simulink model "Model_TranslationEngine64"  (R2022b)
settings: Solver=FixedStepDiscrete  StartTime=0.0  StopTime=5  RelTol=1e-3  EnableMultiTasking=on
InitFcn:
  | % Initialize model
  | ModelSettings=BTConfig.GetModelSettings();
  | 
  | ModelSettings.Validate();
  | 
  | ModelInit;
  | 
  | 
  | % load library data
  | GainLibrary_data;
  | % Load saved values from partition process
  | CapturedConstMask.LoadMapFromFile(bdroot)
StartFcn:
  | % make sure all the simulated RTC requests are found
  | %RTC_SIM_OBJ.ValidateREQs();
undefined symbols (not defined in the file or in its folder): AA, BPLP, Column, NumHFRefBPF, NumHFRefLPF, NumMusicChannels, Row, VolumeMuteConfig
libraries: TuneVar x925, TOP x490, FeaturePath x111, CapturedConstLib x52
(part 19 of 34)

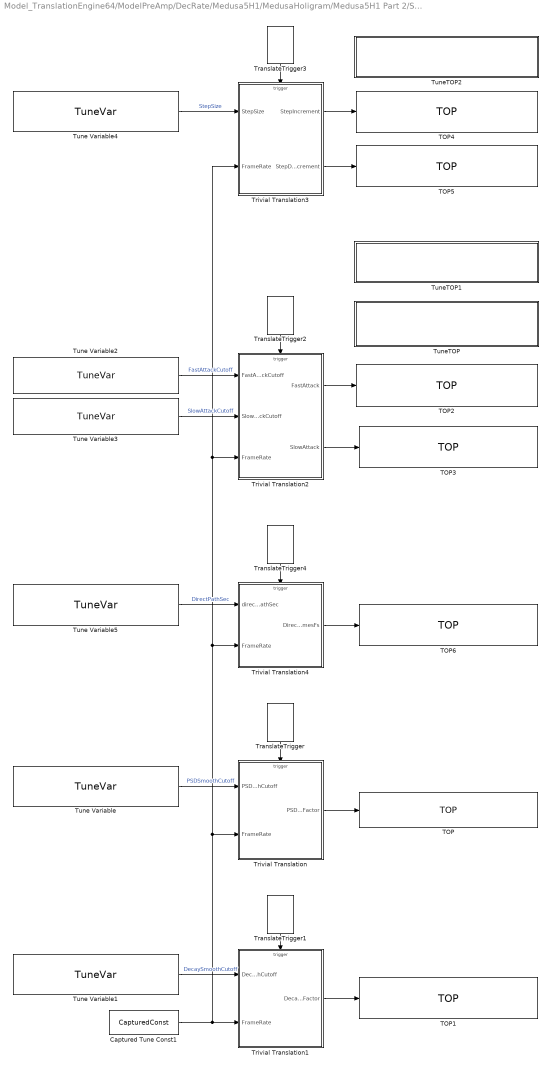
== system Model_TranslationEngine64/ModelPreAmp/DecRate/Medusa5H1/MedusaHoligram/Medusa5H1 Part 2/SPUM Decay Estimate/Decay Estimate ==
  Captured Tune Const1 : CapturedConstLib/CapturedConst  TriggerInit=[-265 -88 -165 -52]  Role=Automatic
      settings: SourceProductName=Bose Talaria
  TOP : TOP/TOP  TriggerInit=[100 -405 360 -355]  TopName=PSDSmoothFactor  DataTypeOut=single  BankNumber=0  PreOverlay=false  PostOverlay=false  Role=Automatic
      settings: SourceProductName=Bose Talaria
  TOP1 : TOP/TOP  TriggerInit=[100 -135 360 -75]  TopName=DecaySmoothFactor  DataTypeOut=single  BankNumber=0  PreOverlay=false  PostOverlay=false  Role=Automatic
      settings: SourceProductName=Bose Talaria
  TOP2 : TOP/TOP  TriggerInit=[95 -1030 360 -970]  TopName=FastAttack  DataTypeOut=single  BankNumber=0  PreOverlay=false  PostOverlay=false  Role=Automatic
      settings: SourceProductName=Bose Talaria
  TOP3 : TOP/TOP  TriggerInit=[100 -940 360 -880]  TopName=SlowAttack  DataTypeOut=single  BankNumber=0  PreOverlay=false  PostOverlay=false  Role=Automatic
      settings: SourceProductName=Bose Talaria
  TOP4 : TOP/TOP  TriggerInit=[95 -1430 360 -1370]  TopName=StepIncrement  DataTypeOut=single  BankNumber=0  PreOverlay=false  PostOverlay=false  Role=Automatic
      settings: SourceProductName=Bose Talaria
  TOP5 : TOP/TOP  TriggerInit=[95 -1350 360 -1290]  TopName=StepDecrement  DataTypeOut=single  BankNumber=0  PreOverlay=false  PostOverlay=false  Role=Automatic
      settings: SourceProductName=Bose Talaria
  TOP6 : TOP/TOP  TriggerInit=[100 -680 360 -620]  TopName=DirectPathFramesFs  DataTypeOut=single  BankNumber=0  PreOverlay=false  PostOverlay=false  Role=Automatic
      settings: SourceProductName=Bose Talaria
  TranslateTrigger : TuneVar/TranslateTrigger  TriggerInit=[-34 -535 4 -480]
      settings: SourceProductName=Bose Talaria
  TranslateTrigger1 : TuneVar/TranslateTrigger  TriggerInit=[-34 -255 4 -200]
      settings: SourceProductName=Bose Talaria
  TranslateTrigger2 : TuneVar/TranslateTrigger  TriggerInit=[-34 -1130 4 -1075]
      settings: SourceProductName=Bose Talaria
  TranslateTrigger3 : TuneVar/TranslateTrigger  TriggerInit=[-34 -1525 4 -1470]
      settings: SourceProductName=Bose Talaria
  TranslateTrigger4 : TuneVar/TranslateTrigger  TriggerInit=[-34 -795 4 -740]
      settings: SourceProductName=Bose Talaria
  Trivial Translation : MATLAB Function  TreatAsAtomicUnit=on
  Trivial Translation1 : MATLAB Function  TreatAsAtomicUnit=on
  Trivial Translation2 : MATLAB Function  TreatAsAtomicUnit=on
  Trivial Translation3 : MATLAB Function  TreatAsAtomicUnit=on
  Trivial Translation4 : MATLAB Function  TreatAsAtomicUnit=on
  Tune Variable : TuneVar/TuneVar  Description=Cutoff frequency for single pole averager that smooths energy sequence for decay estimation.  TuneName=PSDSmoothCutoff  SpecifyMaxSize=off  VariableDim=1 (Row)  MaxSize=[1 1]  TunabilityNumber=2  MinValue=[]  MaxValue=[]  TriggerInit=[-405 -444 -165 -386]  MaskValue=3.890381009312922
      settings: SourceProductName=Bose Talaria
  Tune Variable1 : TuneVar/TuneVar  Description=Cutoff frequency for single pole averager that further smooths decay.  TuneName=DecaySmoothCutoff  SpecifyMaxSize=off  VariableDim=1 (Row)  MaxSize=[1 1]  TunabilityNumber=2  MinValue=[]  MaxValue=[]  TriggerInit=[-405 -169 -165 -111]  MaskValue=0.13777233653605728
      settings: SourceProductName=Bose Talaria
  Tune Variable2 : TuneVar/TuneVar  Description=Cutoff frequency for single pole averager when decay parameter is increasing.  TuneName=FastAttackCutoff  SpecifyMaxSize=off  VariableDim=1 (Row)  MaxSize=[1 1]  TunabilityNumber=2  MinValue=[]  MaxValue=[]  TriggerInit=[-405 -1041 -165 -989]  MaskValue=8.8214110578435392
      settings: SourceProductName=Bose Talaria
  Tune Variable3 : TuneVar/TuneVar  Description=Cutoff frequency for single pole averager when decay parameter is decreasing (slow decay).  TuneName=SlowAttackCutoff  SpecifyMaxSize=off  VariableDim=1 (Row)  MaxSize=[1 1]  TunabilityNumber=2  MinValue=[]  MaxValue=[]  TriggerInit=[-405 -981 -165 -929]  MaskValue=0.27692922573026191
      settings: SourceProductName=Bose Talaria
  Tune Variable4 : TuneVar/TuneVar  Description=Step size for decay slewing.  TuneName=StepSize  SpecifyMaxSize=off  VariableDim=1 (Row)  MaxSize=[1 1]  TunabilityNumber=1  MinValue=[]  MaxValue=[]  TriggerInit=[-405 -1429 -165 -1371]  MaskValue=2
      settings: SourceProductName=Bose Talaria
  Tune Variable5 : TuneVar/TuneVar  Description=This is the time in seconds that separates dry (or direct) and reverb parts. The larger directPathSec becomes, the more energy goes into the “impulse” because a longer period of time past “onset” is considered direct energy. Ideally this value is equivalent to an integer multiple of a frame period.  TuneName=DirectPathSec  SpecifyMaxSize=off  VariableDim=1 (Row)  MaxSize=[1 1]  TunabilityNumber=2  MinValue=[]  MaxValue=[]  TriggerInit=[-405 -710 -165 -650]  MaskValue=0.023219954648526078
      settings: SourceProductName=Bose Talaria
  TuneTOP : Subsystem  Description=Prevent spurious change in slope estimation. Signal energy must overcome the noise floor before we accept current derivative as slope of the decay.  mask(Talaria Trivial Tune TOP){TriggerInit=[95 -1121 360 -1059], TopName=NoiseFloor, TuneName=NoiseFloor, DataTypeOut=single, MaskValue=3, TunabilityNumber=2, MinValue=[], MaxValue=[], BankNumber=0, PreOverlay=false, PostOverlay=false, UseSameName=on}
      mask prompts: TriggerInit "Hidden: MoveFcn redraw"; TopName "Name:"; TuneName "Name of TuneVar:"; DataTypeOut "Data type:"; MaskValue "Default Value:"; TunabilityNumber "Tunability:"; MinValue "Min Value:"; MaxValue "Max Value:"; BankNumber "Target memory bank number:"; PreOverlay "Requires pre-overlay action:"; PostOverlay "Requires post-overlay action:"; UseSameName "Use same name for tune variable and TOP"
      mask help: The TuneTOP block encapsultes a Target Overlay Parameter, a Tune Variable, and a Trivial Translation between them.
      mask init:
      | [ok,activeTopPath,activeTunePath] = TuneTOP_Mask.Init(gcbh);
      settings: MoveFcn=TuneTOP_Mask.CB_TriggerInit(gcbh);
      mask Callback TriggerInit: TuneTOP_Mask.CB_TriggerInit(gcbh);
      mask TypeOptions TopName: TOP/TopName
      mask TypeOptions TuneName: Tune Variable/TuneName
      mask TypeOptions DataTypeOut: TOP/DataTypeOut
      mask TypeOptions MaskValue: Tune Variable/MaskValue
      mask TypeOptions TunabilityNumber: Tune Variable/TunabilityNumber
      mask Callback TunabilityNumber: TuneVarMask.CB_TunabilityNumber(gcbh);
      mask TypeOptions MinValue: Tune Variable/MinValue
      mask TypeOptions MaxValue: Tune Variable/MaxValue
      mask TypeOptions BankNumber: TOP/BankNumber
      mask TypeOptions PreOverlay: TOP/PreOverlay
      mask TypeOptions PostOverlay: TOP/PostOverlay
      mask Callback UseSameName: TuneTOP_Mask.CB_UseSameName(gcbh);
      mask DialogControl toolPanel Prompt: Tuning Tool Hints
      mask DialogControl DescriptionGroup Prompt: Description
      mask DialogControl EditDescription Prompt: Edit Description
      mask DialogControl EditDescription Callback: TuneTOP_Mask.CB_EditDescription(gcbh);
      mask DialogControl TunabilityText Prompt: Easy: Changes nearly every tuning.
      mask DialogControl AdvancedPanel Prompt: Advanced
      mask DialogControl ConvertToFullTranslation Prompt: Irreversible conversion to full translation
      mask DialogControl ConvertToFullTranslation Callback: TuneTOP_Mask.CB_ConvertToFullTranslation(gcbh);
      mask DialogControl ErrorContainer Prompt: Error Messages
      mask Display:
      | % retrieve icon definition
      | [path,w,h] = TuneTOP_Mask.Icon();
      | 
      | % retrieve the block's pixel size
      | pos = get(gcbh,'position');
      | bw = pos(3) - pos(1);
      | bh = pos(4) - pos(2);
      | 
      | % draw centered icon
      | xAdj = bw/2 - w/2 + 5;
      | yAdj = bh/2 - h/2 + 4;
      | for i=1:length(path)
      | 	patch(path(i).x+xAdj, path(i).y+yAdj, path(i).rgb);
      | end
      | 
      | % show the top name or an X
      | if (exist('ok','var') && ok)
      | 	text(bw*0.5, bh*0.2, activeTopPath, 'horizontalAlignment', 'center');
      | 	patch(0,0,[1 1 1]);
      | 	patch(bw,bh,[1 1 1]);
      | else
      | 	tx=bw*0.03;
      | 	ty=bh*0.03;
      | 	patch([0 tx bw bw-tx], [ty 0 bh-ty bh], [1 0 0]);
      | 	patch([0 bw-tx bw tx], [bh-ty 0 ty bh], [1 0 0]);
      | end
  TuneTOP1 : Subsystem  Description=Thresold for detecting an onset strike.  mask(Talaria Trivial Tune TOP){TriggerInit=[95 -1208 360 -1152], TopName=OnsetThreshold, TuneName=OnsetThreshold, DataTypeOut=single, MaskValue=1.875, TunabilityNumber=2, MinValue=[], MaxValue=[], BankNumber=0, PreOverlay=false, PostOverlay=false, UseSameName=on}
      mask prompts: TriggerInit "Hidden: MoveFcn redraw"; TopName "Name:"; TuneName "Name of TuneVar:"; DataTypeOut "Data type:"; MaskValue "Default Value:"; TunabilityNumber "Tunability:"; MinValue "Min Value:"; MaxValue "Max Value:"; BankNumber "Target memory bank number:"; PreOverlay "Requires pre-overlay action:"; PostOverlay "Requires post-overlay action:"; UseSameName "Use same name for tune variable and TOP"
      mask help: The TuneTOP block encapsultes a Target Overlay Parameter, a Tune Variable, and a Trivial Translation between them.
      mask init:
      | [ok,activeTopPath,activeTunePath] = TuneTOP_Mask.Init(gcbh);
      settings: MoveFcn=TuneTOP_Mask.CB_TriggerInit(gcbh);
      mask Callback TriggerInit: TuneTOP_Mask.CB_TriggerInit(gcbh);
      mask TypeOptions TopName: TOP/TopName
      mask TypeOptions TuneName: Tune Variable/TuneName
      mask TypeOptions DataTypeOut: TOP/DataTypeOut
      mask TypeOptions MaskValue: Tune Variable/MaskValue
      mask TypeOptions TunabilityNumber: Tune Variable/TunabilityNumber
      mask Callback TunabilityNumber: TuneVarMask.CB_TunabilityNumber(gcbh);
      mask TypeOptions MinValue: Tune Variable/MinValue
      mask TypeOptions MaxValue: Tune Variable/MaxValue
      mask TypeOptions BankNumber: TOP/BankNumber
      mask TypeOptions PreOverlay: TOP/PreOverlay
      mask TypeOptions PostOverlay: TOP/PostOverlay
      mask Callback UseSameName: TuneTOP_Mask.CB_UseSameName(gcbh);
      mask DialogControl toolPanel Prompt: Tuning Tool Hints
      mask DialogControl DescriptionGroup Prompt: Description
      mask DialogControl EditDescription Prompt: Edit Description
      mask DialogControl EditDescription Callback: TuneTOP_Mask.CB_EditDescription(gcbh);
      mask DialogControl TunabilityText Prompt: Easy: Changes nearly every tuning.
      mask DialogControl AdvancedPanel Prompt: Advanced
      mask DialogControl ConvertToFullTranslation Prompt: Irreversible conversion to full translation
      mask DialogControl ConvertToFullTranslation Callback: TuneTOP_Mask.CB_ConvertToFullTranslation(gcbh);
      mask DialogControl ErrorContainer Prompt: Error Messages
      mask Display:
      | % retrieve icon definition
      | [path,w,h] = TuneTOP_Mask.Icon();
      | 
      | % retrieve the block's pixel size
      | pos = get(gcbh,'position');
      | bw = pos(3) - pos(1);
      | bh = pos(4) - pos(2);
      | 
      | % draw centered icon
      | xAdj = bw/2 - w/2 + 5;
      | yAdj = bh/2 - h/2 + 4;
      | for i=1:length(path)
      | 	patch(path(i).x+xAdj, path(i).y+yAdj, path(i).rgb);
      | end
      | 
      | % show the top name or an X
      | if (exist('ok','var') && ok)
      | 	text(bw*0.5, bh*0.2, activeTopPath, 'horizontalAlignment', 'center');
      | 	patch(0,0,[1 1 1]);
      | 	patch(bw,bh,[1 1 1]);
      | else
      | 	tx=bw*0.03;
      | 	ty=bh*0.03;
      | 	patch([0 tx bw bw-tx], [ty 0 bh-ty bh], [1 0 0]);
      | 	patch([0 bw-tx bw tx], [bh-ty 0 ty bh], [1 0 0]);
      | end
  TuneTOP2 : Subsystem  Description=Threshold to accept change in decay.  mask(Talaria Trivial Tune TOP){TriggerInit=[95 -1508 360 -1452], TopName=SlewThreshold, TuneName=SlewThreshold, DataTypeOut=single, MaskValue=0.8, TunabilityNumber=2, MinValue=[], MaxValue=[], BankNumber=0, PreOverlay=false, PostOverlay=false, UseSameName=on}
      mask prompts: TriggerInit "Hidden: MoveFcn redraw"; TopName "Name:"; TuneName "Name of TuneVar:"; DataTypeOut "Data type:"; MaskValue "Default Value:"; TunabilityNumber "Tunability:"; MinValue "Min Value:"; MaxValue "Max Value:"; BankNumber "Target memory bank number:"; PreOverlay "Requires pre-overlay action:"; PostOverlay "Requires post-overlay action:"; UseSameName "Use same name for tune variable and TOP"
      mask help: The TuneTOP block encapsultes a Target Overlay Parameter, a Tune Variable, and a Trivial Translation between them.
      mask init:
      | [ok,activeTopPath,activeTunePath] = TuneTOP_Mask.Init(gcbh);
      settings: MoveFcn=TuneTOP_Mask.CB_TriggerInit(gcbh);
      mask Callback TriggerInit: TuneTOP_Mask.CB_TriggerInit(gcbh);
      mask TypeOptions TopName: TOP/TopName
      mask TypeOptions TuneName: Tune Variable/TuneName
      mask TypeOptions DataTypeOut: TOP/DataTypeOut
      mask TypeOptions MaskValue: Tune Variable/MaskValue
      mask TypeOptions TunabilityNumber: Tune Variable/TunabilityNumber
      mask Callback TunabilityNumber: TuneVarMask.CB_TunabilityNumber(gcbh);
      mask TypeOptions MinValue: Tune Variable/MinValue
      mask TypeOptions MaxValue: Tune Variable/MaxValue
      mask TypeOptions BankNumber: TOP/BankNumber
      mask TypeOptions PreOverlay: TOP/PreOverlay
      mask TypeOptions PostOverlay: TOP/PostOverlay
      mask Callback UseSameName: TuneTOP_Mask.CB_UseSameName(gcbh);
      mask DialogControl toolPanel Prompt: Tuning Tool Hints
      mask DialogControl DescriptionGroup Prompt: Description
      mask DialogControl EditDescription Prompt: Edit Description
      mask DialogControl EditDescription Callback: TuneTOP_Mask.CB_EditDescription(gcbh);
      mask DialogControl TunabilityText Prompt: Easy: Changes nearly every tuning.
      mask DialogControl AdvancedPanel Prompt: Advanced
      mask DialogControl ConvertToFullTranslation Prompt: Irreversible conversion to full translation
      mask DialogControl ConvertToFullTranslation Callback: TuneTOP_Mask.CB_ConvertToFullTranslation(gcbh);
      mask DialogControl ErrorContainer Prompt: Error Messages
      mask Display:
      | % retrieve icon definition
      | [path,w,h] = TuneTOP_Mask.Icon();
      | 
      | % retrieve the block's pixel size
      | pos = get(gcbh,'position');
      | bw = pos(3) - pos(1);
      | bh = pos(4) - pos(2);
      | 
      | % draw centered icon
      | xAdj = bw/2 - w/2 + 5;
      | yAdj = bh/2 - h/2 + 4;
      | for i=1:length(path)
      | 	patch(path(i).x+xAdj, path(i).y+yAdj, path(i).rgb);
      | end
      | 
      | % show the top name or an X
      | if (exist('ok','var') && ok)
      | 	text(bw*0.5, bh*0.2, activeTopPath, 'horizontalAlignment', 'center');
      | 	patch(0,0,[1 1 1]);
      | 	patch(bw,bh,[1 1 1]);
      | else
      | 	tx=bw*0.03;
      | 	ty=bh*0.03;
      | 	patch([0 tx bw bw-tx], [ty 0 bh-ty bh], [1 0 0]);
      | 	patch([0 bw-tx bw tx], [bh-ty 0 ty bh], [1 0 0]);
      | end
  wires:
  Trivial Translation3/2(StepDecrement) -> TOP5/1
  Trivial Translation3/1(StepIncrement) -> TOP4/1
  Tune Variable4/1 -> Trivial Translation3/1(StepSize)  "StepSize"
  TranslateTrigger3/1 -> Trivial Translation3/Trigger
  Trivial Translation2/2(SlowAttack) -> TOP3/1
  Tune Variable3/1 -> Trivial Translation2/2(SlowAttackCutoff)  "SlowAttackCutoff"
  Tune Variable2/1 -> Trivial Translation2/1(FastAttackCutoff)  "FastAttackCutoff"
  TranslateTrigger2/1 -> Trivial Translation2/Trigger
  Trivial Translation2/1(FastAttack) -> TOP2/1
  Tune Variable1/1 -> Trivial Translation1/1(DecaySmoothCutoff)  "DecaySmoothCutoff"
  TranslateTrigger1/1 -> Trivial Translation1/Trigger
  Trivial Translation1/1(DecaySmoothFactor) -> TOP1/1
  Trivial Translation/1(PSDSmoothFactor) -> TOP/1
  TranslateTrigger/1 -> Trivial Translation/Trigger
  Tune Variable/1 -> Trivial Translation/1(PSDSmoothCutoff)  "PSDSmoothCutoff"
  TranslateTrigger4/1 -> Trivial Translation4/Trigger
  Trivial Translation4/1(DirectPathFramesFs) -> TOP6/1
  Tune Variable5/1 -> Trivial Translation4/1(directPathSec)  "DirectPathSec"
  Captured Tune Const1/1 -> Trivial Translation1/2(FrameRate), Trivial Translation3/2(FrameRate), Trivial Translation2/3(FrameRate), Trivial Translation4/2(FrameRate), Trivial Translation/2(FrameRate)

== system Model_TranslationEngine64/ModelPreAmp/DecRate/Medusa5H1/MedusaHoligram/Medusa5H1 Part 2/SPUM Decay Estimate/High-pass filter > 6kHz ==
  InnerLink : Subsystem  mask(Bose Pool IIR Tunable){FeatureName=HPF, Config=InnerLinkConfig}
      mask prompts: FeatureName "Filter name/purpose"; Config "PoolIirTunableConfig"
      mask help:
      | Pool IIR Tunable is a configurable multi-channel IIR filter that supports one or more channels. This block offers flexibility of tuning the number of stages and coefficients. Different filter coefficients and number of stages (biquads) can be used for each channel filter. The Pool IIR Tunable block supports different implementations, which could be configured at build-time:
      |
      | (i)   Generic: IIR filter code not optimized for any processor
      | (ii)  SharcCore: IIR filters executing on core (uses pooliir.asm CRL)
      | (iii) SharcGulAccel: IIR filters executing on IIR hardware accelerator, offloading MIPS usage from core
      | (iv) SharcGxpAccel: IIR filters take advantage of additional accelerators available on GXP processor
      | (v)  Hexagon: TBD
      |
      | NOTE: When using Pool IIR for Sharc-plus based processors, the codeWorkMemory buffer and input buffer should always be mapped to L1 memory to optimize MIPS utilization and avoid audio artifacts.
      |
      | For more information, please see 'Help'.
      mask init:
      | blkh=gcbh;
      | Config=BTConfig.Assert(blkh,Config);
      | 
      | Config.Validate();
      | Config.DoMaskInit(blkh);
      mask Help:
      | <b>Input signals: </b>
      | AudioIn: input channels [frame size x number of channels]
      | 
      | <b>Output signals: </b>
      | AudioOut: output channels [frame size x number of channels]
      | 
      | <b>Mask parameters: </b>
      | PoolIirTunableConfig
      | Filter name/purpose
      mask TypeOptions FeatureName: PoolIirTunableWithReset/FeatureName
      mask Display: DrawPoolIirIcon;

== system Model_TranslationEngine64/ModelPreAmp/DecRate/Medusa5H1/MedusaHoligram/Medusa5H1 Part 3/On/Delay Tuning ==
  Delay Translation : Subsystem  mask(Alignment Delay Translation){Config=ConfigBTC.AlignmentDelayTranslation}
      mask prompts: Config "MedusaAlignmentDelayTranslationConfig"
      mask help: This block accepts Wiggle Delay and Holigram Filter Delay and outputs all Medusa fixed alignment delay amounts in samples.
      mask init:
      | blkh=gcbh;
      | Config=BTConfig.Assert(blkh,Config);
      | 
      | Config.Validate();
  Tune Variable : TuneVar/TuneVar  TuneName=DeciRateWiggleFilterDelaySamples1  SpecifyMaxSize=off  VariableDim=1 (Row)  MaxSize=[1 1]  TunabilityNumber=1  MinValue=[]  MaxValue=[]  TriggerInit=[-115 25 55 75]  MaskValue=ConfigBTC.AlignmentDelayTranslation.DefaultTuning.DeciRateWiggleDelay
      settings: SourceProductName=Bose Talaria
  Tune Variable1 : TuneVar/TuneVar  TuneName=DeciRateNearWiggleFilterDelaySamples1  SpecifyMaxSize=off  VariableDim=1 (Row)  MaxSize=[1 1]  TunabilityNumber=1  MinValue=[]  MaxValue=[]  TriggerInit=[-115 87 55 133]  MaskValue=ConfigBTC.AlignmentDelayTranslation.DefaultTuning.DeciRateNearWiggleDelay
      settings: SourceProductName=Bose Talaria
  wires:
  Tune Variable1/1 -> Delay Translation/2(DeciRateNearWiggleDelaySamples)  "DeciRateNearWiggleFilterDelaySamples1"
  Tune Variable/1 -> Delay Translation/1(DeciRateWiggleDelaySamples)  "DeciRateWiggleFilterDelaySamples1"

== system Model_TranslationEngine64/ModelPreAmp/DecRate/Medusa5H1/MedusaHoligram/Medusa5H1 Part 3/On/Expand Tail Components ==
  Tail Component EQ : Subsystem  LoadFcn="fprintf(\"\\n ''%s'' block does not support BTC and hence, it will be deprecated soon. Please replace all the active instances of \"\"PooliirwithNonTrivialTranslations\"\" with an equivalent BTC block.\", gcb);"  mask(Bose Pool IIR){maxNumStages=config.tailCompEQ.maxNumStages, numStages=config.tailCompEQ.numStages, sosCoefficients=config.tailCompEQ.coeffs, alias='Default', variantType='Hexagon', FeatureName=tailCompEQ}
      mask prompts: maxNumStages "Maximum number of stages"; numStages "Number of stages per channel"; sosCoefficients "Coefficient pool"; variantType "Variant"; FeatureName "Filter name/purpose"
      mask init: same as Model_TranslationEngine64/ModelPreAmp/DecRate/AudioPilot35/EntertainmentLevelDetection/PreProcessing/PreEmphasisShelfFilter
      mask TypeOptions FeatureName: InnerLink/FeatureName
      mask Display:
      | [path,w,h] = IconIIR_Mask();
      | 
      | % work in pixels since the icon does not scale
      | pos = get(gcbh,'position');
      | bw = pos(3) - pos(1);
      | bh = pos(4) - pos(2);
      | 
      | % Draw centered icon
      | xAdj = bw/2 - w/2;
      | yAdj = bh/2 - h/2 + 4;
      | for i=1:length(path)
      | %     patch(path(i).x+xAdj, path(i).y+yAdj, path(i).rgb);
      |     plot(path(i).x+xAdj, path(i).y+yAdj);
      | end
      | 
      | % Anchor the corners of the coordinate system
      | patch(0,0,[1 1 1]);
      | patch(bw,bh,[1 1 1]);
      | 
      | % Display some text
      | text(bw/2, 1,'Pool IIR', ...
      |     'horizontalAlignment','center', ...
      |     'VerticalAlignment','bottom');
  TuneTOP : Subsystem  mask(Talaria Trivial Tune TOP){TriggerInit=[265 167 435 223], TopName=WiggleFilter, TuneName=WiggleFilter, DataTypeOut=single, MaskValue=config.wiggleFilterDefault, TunabilityNumber=1, MinValue=[], MaxValue=[], BankNumber=0, PreOverlay=false, PostOverlay=false, UseSameName=on}
      mask prompts: TriggerInit "Hidden: MoveFcn redraw"; TopName "Name:"; TuneName "Name of TuneVar:"; DataTypeOut "Data type:"; MaskValue "Default Value:"; TunabilityNumber "Tunability:"; MinValue "Min Value:"; MaxValue "Max Value:"; BankNumber "Target memory bank number:"; PreOverlay "Requires pre-overlay action:"; PostOverlay "Requires post-overlay action:"; UseSameName "Use same name for tune variable and TOP"
      mask help: The TuneTOP block encapsultes a Target Overlay Parameter, a Tune Variable, and a Trivial Translation between them.
      mask init:
      | [ok,activeTopPath,activeTunePath] = TuneTOP_Mask.Init(gcbh);
      settings: MoveFcn=TuneTOP_Mask.CB_TriggerInit(gcbh);
      mask Callback TriggerInit: TuneTOP_Mask.CB_TriggerInit(gcbh);
      mask TypeOptions TopName: TOP/TopName
      mask TypeOptions TuneName: Tune Variable/TuneName
      mask TypeOptions DataTypeOut: TOP/DataTypeOut
      mask TypeOptions MaskValue: Tune Variable/MaskValue
      mask TypeOptions TunabilityNumber: Tune Variable/TunabilityNumber
      mask Callback TunabilityNumber: TuneVarMask.CB_TunabilityNumber(gcbh);
      mask TypeOptions MinValue: Tune Variable/MinValue
      mask TypeOptions MaxValue: Tune Variable/MaxValue
      mask TypeOptions BankNumber: TOP/BankNumber
      mask TypeOptions PreOverlay: TOP/PreOverlay
      mask TypeOptions PostOverlay: TOP/PostOverlay
      mask Callback UseSameName: TuneTOP_Mask.CB_UseSameName(gcbh);
      mask DialogControl toolPanel Prompt: Tuning Tool Hints
      mask DialogControl DescriptionGroup Prompt: Description
      mask DialogControl EditDescription Prompt: Edit Description
      mask DialogControl EditDescription Callback: TuneTOP_Mask.CB_EditDescription(gcbh);
      mask DialogControl TunabilityText Prompt: Easy: Changes nearly every tuning.
      mask DialogControl AdvancedPanel Prompt: Advanced
      mask DialogControl ConvertToFullTranslation Prompt: Irreversible conversion to full translation
      mask DialogControl ConvertToFullTranslation Callback: TuneTOP_Mask.CB_ConvertToFullTranslation(gcbh);
      mask DialogControl ErrorContainer Prompt: Error Messages
      mask DialogControl ErrorText Prompt: Default value cannot be empty. Tune variables must have non-zero dimensions.
      mask Display:
      | % retrieve icon definition
      | [path,w,h] = TuneTOP_Mask.Icon();
      | 
      | % retrieve the block's pixel size
      | pos = get(gcbh,'position');
      | bw = pos(3) - pos(1);
      | bh = pos(4) - pos(2);
      | 
      | % draw centered icon
      | xAdj = bw/2 - w/2 + 5;
      | yAdj = bh/2 - h/2 + 4;
      | for i=1:length(path)
      | 	patch(path(i).x+xAdj, path(i).y+yAdj, path(i).rgb);
      | end
      | 
      | % show the top name or an X
      | if (exist('ok','var') && ok)
      | 	text(bw*0.5, bh*0.2, activeTopPath, 'horizontalAlignment', 'center');
      | 	patch(0,0,[1 1 1]);
      | 	patch(bw,bh,[1 1 1]);
      | else
      | 	tx=bw*0.03;
      | 	ty=bh*0.03;
      | 	patch([0 tx bw bw-tx], [ty 0 bh-ty bh], [1 0 0]);
      | 	patch([0 bw-tx bw tx], [bh-ty 0 ty bh], [1 0 0]);
      | end

== system Model_TranslationEngine64/ModelPreAmp/DecRate/Medusa5H1/MedusaHoligram/Medusa5H1 Part 3/On/Full-rate Mixer ==
  Full-Rate Mixer with CAE & Fade Ramper : Subsystem  mask{MedusaFRMConfig=config.FRMConfig, MedusaFRMTune=config.FRMTune}
      mask prompts: MedusaFRMConfig "Config struct name:"; MedusaFRMTune "Tune struct name:"
      mask init:
      | %MedusaConfig = generateMedusaConfig(system_definitions);
      | 
      | % Initialize model parameters
      | %MedusaFullRateMixerInit(MedusaConfig);

== system Model_TranslationEngine64/ModelPreAmp/DecRate/Medusa5H1/MedusaHoligram/Medusa5H1 Part 3/On/Premix ==
  Premix with Mono-Surround & CAE with Fade Ramper : Subsystem  mask(Medusa Premix 5H){MedusaPremixConfig=config.PremixConfig, MedusaPremixTune=config.PremixTune, MSConfig=config.MSConfig}
      mask prompts: MedusaPremixConfig "Config struct name:"; MedusaPremixTune "Tune struct name:"; MSConfig "Mono-Surround Config:"
      mask init:
      | % RTC_SIM_OBJ = RTC_SimData();
      | 
      | % MedusaConfig = generateMedusaConfig(system_definitions);
      | 
      | % Initialize model parameters
      | % MedusaPremixExampleInit(MedusaConfig);
      settings: LibrarySourceBlock=MedusaPremix/Premix with Mono-Surround & CAE with Fade Ramper

== system Model_TranslationEngine64/ModelPreAmp/DecRate/Medusa5H1/MedusaHoligram/Medusa5H1 Part 3/On/VLS Gains Computation ==
  VLS Gains Drv : Subsystem  mask(VLS Gains){configStruct=vlsConfigStruct.VLSGainsConfig, tuneStruct=vlsConfigStruct.VLSGainsTune, FeatureName=VLSDrvGains}
      mask prompts: configStruct "Config struct name:"; tuneStruct "Tune struct name:"; FeatureName "FeaturePath name:"
      mask init:
      | VLSGainsMaskInit(gcbh, FeatureName);
      mask TypeOptions FeatureName: FeaturePath/FeatureName
  VLS Gains Pax : Subsystem  mask(VLS Gains){configStruct=vlsConfigStruct.VLSGainsConfig, tuneStruct=vlsConfigStruct.VLSGainsTune, FeatureName=VLSPaxGains}
      mask prompts: configStruct "Config struct name:"; tuneStruct "Tune struct name:"; FeatureName "FeaturePath name:"
      mask init:
      | VLSGainsMaskInit(gcbh, FeatureName);
      mask TypeOptions FeatureName: FeaturePath/FeatureName

== system Model_TranslationEngine64/ModelPreAmp/DecRate/Medusa5H1/MedusaHoligram/Medusa5H1 Part 4/On/DR Mix Matrix with Hybrid Holigram EQ ==
  FeaturePath : FeaturePath/FeaturePath  FeatureName=DRHoligram  IsGroup=off  GroupNumber=-1  IsModule=off  TriggerInit=[375 434 490 541]
      settings: SourceProductName=Bose Talaria
  IIR : Subsystem  mask(Bose Pool IIR Tunable){FeatureName=PoolIirTunableConfig, Config=Config.Iir}
      mask prompts: FeatureName "Filter name/purpose"; Config "PoolIirTunableConfig"
      mask help:
      | Pool IIR Tunable is a configurable multi-channel IIR filter that supports one or more channels. This block offers flexibility of tuning the number of stages and coefficients. Different filter coefficients and number of stages (biquads) can be used for each channel filter. The Pool IIR Tunable block supports different implementations, which could be configured at build-time:
      |
      | (i)   Generic: IIR filter code not optimized for any processor
      | (ii)  SharcCore: IIR filters executing on core (uses pooliir.asm CRL)
      | (iii) SharcGulAccel: IIR filters executing on IIR hardware accelerator, offloading MIPS usage from core
      | (iv) SharcGxpAccel: IIR filters take advantage of additional accelerators available on GXP processor
      | (v)  Hexagon: TBD
      |
      | NOTE: When using Pool IIR for Sharc-plus based processors, the codeWorkMemory buffer and input buffer should always be mapped to L1 memory to optimize MIPS utilization and avoid audio artifacts.
      |
      | For more information, please see 'Help'.
      mask init:
      | blkh=gcbh;
      | Config=BTConfig.Assert(blkh,Config);
      | 
      | Config.Validate();
      | Config.DoMaskInit(blkh);
      mask Help:
      | <b>Input signals: </b>
      | AudioIn: input channels [frame size x number of channels]
      | 
      | <b>Output signals: </b>
      | AudioOut: output channels [frame size x number of channels]
      | 
      | <b>Mask parameters: </b>
      | PoolIirTunableConfig
      | Filter name/purpose
      mask TypeOptions FeatureName: PoolIirTunableWithReset/FeatureName
      mask Display: DrawPoolIirIcon;
  Tune Translations : Subsystem

== system Model_TranslationEngine64/ModelPreAmp/DecRate/Medusa5H1/MedusaHoligram/Medusa5H1 Part 4/On/FR IIR Holigram EQ ==
  FeaturePath : FeaturePath/FeaturePath  FeatureName=FRHoligram  IsGroup=off  GroupNumber=-1  IsModule=off  TriggerInit=[225 439 340 546]
      settings: SourceProductName=Bose Talaria
  IIR : Subsystem  mask(Bose Pool IIR Tunable){FeatureName=IirConfig, Config=IirConfig}
      mask prompts: FeatureName "Filter name/purpose"; Config "PoolIirTunableConfig"
      mask help:
      | Pool IIR Tunable is a configurable multi-channel IIR filter that supports one or more channels. This block offers flexibility of tuning the number of stages and coefficients. Different filter coefficients and number of stages (biquads) can be used for each channel filter. The Pool IIR Tunable block supports different implementations, which could be configured at build-time:
      |
      | (i)   Generic: IIR filter code not optimized for any processor
      | (ii)  SharcCore: IIR filters executing on core (uses pooliir.asm CRL)
      | (iii) SharcGulAccel: IIR filters executing on IIR hardware accelerator, offloading MIPS usage from core
      | (iv) SharcGxpAccel: IIR filters take advantage of additional accelerators available on GXP processor
      | (v)  Hexagon: TBD
      |
      | NOTE: When using Pool IIR for Sharc-plus based processors, the codeWorkMemory buffer and input buffer should always be mapped to L1 memory to optimize MIPS utilization and avoid audio artifacts.
      |
      | For more information, please see 'Help'.
      mask init:
      | blkh=gcbh;
      | Config=BTConfig.Assert(blkh,Config);
      | 
      | Config.Validate();
      | Config.DoMaskInit(blkh);
      mask Help:
      | <b>Input signals: </b>
      | AudioIn: input channels [frame size x number of channels]
      | 
      | <b>Output signals: </b>
      | AudioOut: output channels [frame size x number of channels]
      | 
      | <b>Mask parameters: </b>
      | PoolIirTunableConfig
      | Filter name/purpose
      mask TypeOptions FeatureName: PoolIirTunableWithReset/FeatureName
      mask Display: DrawPoolIirIcon;

== system Model_TranslationEngine64/ModelPreAmp/DecRate/Medusa5H1/MedusaHoligram/Medusa5H1 Part 4/On/Headrest Comp EQ ==
  note: Output reorder:
      | driver components [Lo, Ro, Ls, Rs, Lsr, Rsr],
      | passenger components [Lo, Ro, Ls, Rs, Lsr, Rsr]
  FeaturePath : FeaturePath/FeaturePath  FeatureName=HeadrestCompEQ  IsGroup=off  GroupNumber=-1  IsModule=off  TriggerInit=[175 204 290 311]
      settings: SourceProductName=Bose Talaria
  IIR : Subsystem  mask(Bose Pool IIR Tunable){FeatureName=IirConfig, Config=IirConfig}
      mask prompts: FeatureName "Filter name/purpose"; Config "PoolIirTunableConfig"
      mask help:
      | Pool IIR Tunable is a configurable multi-channel IIR filter that supports one or more channels. This block offers flexibility of tuning the number of stages and coefficients. Different filter coefficients and number of stages (biquads) can be used for each channel filter. The Pool IIR Tunable block supports different implementations, which could be configured at build-time:
      |
      | (i)   Generic: IIR filter code not optimized for any processor
      | (ii)  SharcCore: IIR filters executing on core (uses pooliir.asm CRL)
      | (iii) SharcGulAccel: IIR filters executing on IIR hardware accelerator, offloading MIPS usage from core
      | (iv) SharcGxpAccel: IIR filters take advantage of additional accelerators available on GXP processor
      | (v)  Hexagon: TBD
      |
      | NOTE: When using Pool IIR for Sharc-plus based processors, the codeWorkMemory buffer and input buffer should always be mapped to L1 memory to optimize MIPS utilization and avoid audio artifacts.
      |
      | For more information, please see 'Help'.
      mask init:
      | blkh=gcbh;
      | Config=BTConfig.Assert(blkh,Config);
      | 
      | Config.Validate();
      | Config.DoMaskInit(blkh);
      mask Help:
      | <b>Input signals: </b>
      | AudioIn: input channels [frame size x number of channels]
      | 
      | <b>Output signals: </b>
      | AudioOut: output channels [frame size x number of channels]
      | 
      | <b>Mask parameters: </b>
      | PoolIirTunableConfig
      | Filter name/purpose
      mask TypeOptions FeatureName: PoolIirTunableWithReset/FeatureName
      mask Display: DrawPoolIirIcon;
  TOP : TOP/TOP  TriggerInit=[815 320 985 380]  TopName=FIRCoeffs  DataTypeOut=single  BankNumber=1  PreOverlay=false  PostOverlay=false  Role=Automatic
      settings: SourceProductName=Bose Talaria
  TOP1 : TOP/TOP  TriggerInit=[815 390 985 450]  TopName=FilterLengths  DataTypeOut=uint32  BankNumber=0  PreOverlay=false  PostOverlay=false  Role=Automatic
      settings: SourceProductName=Bose Talaria
  TOP2 : TOP/TOP  TriggerInit=[815 460 985 520]  TopName=PaddedFilterLengths  DataTypeOut=uint32  BankNumber=0  PreOverlay=false  PostOverlay=false  Role=Automatic
      settings: SourceProductName=Bose Talaria
  TranslateTrigger : TuneVar/TranslateTrigger  TriggerInit=[656 230 694 285]
      settings: SourceProductName=Bose Talaria
  Tune Variable : TuneVar/TuneVar  TuneName=FIRCoeffs  SpecifyMaxSize=off  VariableDim=1 (Row)  MaxSize=[firLength*numEQlink 1]  TunabilityNumber=1  MinValue=[]  MaxValue=[]  TriggerInit=[330 325 500 375]  MaskValue=firCoeffsDefault
      settings: SourceProductName=Bose Talaria
  Tune Variable1 : TuneVar/TuneVar  TuneName=FIRLengths  SpecifyMaxSize=off  VariableDim=1 (Row)  MaxSize=[1 1]  TunabilityNumber=1  MinValue=[]  MaxValue=[]  TriggerInit=[330 395 500 445]  MaskValue=firLength*ones(numEQlink,1)
      settings: SourceProductName=Bose Talaria
  Tune Variable2 : TuneVar/TuneVar  TuneName=PaddedFIRLengths  SpecifyMaxSize=off  VariableDim=1 (Row)  MaxSize=[1 1]  TunabilityNumber=1  MinValue=[]  MaxValue=[]  TriggerInit=[330 465 500 515]  MaskValue=firLength*ones(numEQlink,1)
      settings: SourceProductName=Bose Talaria
  translation : MATLAB Function  TreatAsAtomicUnit=on
  wires:
  translation/2(FIRLengths) -> TOP1/1
  Tune Variable1/1 -> translation/2(FIRLengthsIn)  "FIRLengths"
  translation/1(FIRCoeffs) -> TOP/1
  TranslateTrigger/1 -> translation/Trigger
  Tune Variable/1 -> translation/1(FIRCoeffsIn)  "FIRCoeffs"
  Tune Variable2/1 -> translation/3(PaddedFIRLengthsIn)  "PaddedFIRLengths"
  translation/3(PaddedFIRLengths) -> TOP2/1

== system Model_TranslationEngine64/ModelPreAmp/DecRate/Medusa5H1/MedusaHoligram/Medusa5H1 Part 6/Speaker Delay Tune/Output Delay Translation with Headrest ==
  NonHeadrestSpeakerDelaySamples : Inport
  HeadrestDrvSpeakerDelaySamples : Inport  Port=2
  HeadrestPaxSpeakerDelaySamples : Inport  Port=3
  FullRateHoligramDelaySamples : Inport  Port=4
  TranslateTrigger : TuneVar/TranslateTrigger  TriggerInit=[931 -30 969 25]
      settings: SourceProductName=Bose Talaria
  translation : MATLAB Function  TreatAsAtomicUnit=on  mask{DecimationFactor=Config.DecimationFactor, maxFullRateHoligramDelay=Config.MaxFullRateHoligramDelay, maxFullRateSpeakerDelay=Config.MaxFullRateSpeakerDelay, numHeadrestComps=Config.NumHeadrestComps}
  DeciRateSpeakerDelay : Outport
  FullRateSpeakerDelay : Outport  Port=2
  wires:
  translation/2(FRSpkrDelay) -> FullRateSpeakerDelay/1
  HeadrestDrvSpeakerDelaySamples/1 -> translation/2(tuneHRDrvDelaySamples)
  translation/1(DRDelay) -> DeciRateSpeakerDelay/1
  NonHeadrestSpeakerDelaySamples/1 -> translation/1(tuneNonHRDelaySamples)
  FullRateHoligramDelaySamples/1 -> translation/4(tuneFREQDelaySamples)
  HeadrestPaxSpeakerDelaySamples/1 -> translation/3(tuneHRPaxDelaySamples)
  TranslateTrigger/1 -> translation/Trigger

== system Model_TranslationEngine64/ModelPreAmp/DecRate/Medusa5H1/MedusaPostHoligram/MedusaPostHoligram/On/TuneTOP1 ==
  TOP : TOP/TOP  TriggerInit=[440 20 585 80]  TopName=RoutingMap  DataTypeOut=single  BankNumber=BankNumber  PreOverlay=PreOverlay  PostOverlay=PostOverlay  Role=Automatic
      settings: SourceProductName=Bose Talaria
  TrivialTranslation : TuneVar/TrivialTranslation  TriggerInit=[300 28 350 72]
      settings: SourceProductName=Bose Talaria
  Tune Variable : TuneVar/TuneVar  TuneName=RoutingMap  SpecifyMaxSize=off  VariableDim=1 (Row)  MaxSize=[1 1]  TunabilityNumber=1  MinValue=MinValue  MaxValue=MaxValue  TriggerInit=[20 25 190 75]  MaskValue=MaskValue
      settings: SourceProductName=Bose Talaria
  wires:
  Tune Variable/1 -> TrivialTranslation/1  "RoutingMap"
  TrivialTranslation/1 -> TOP/1

== system Model_TranslationEngine64/ModelPreAmp/DecRate/Medusa5H1/NearWiggleFilters/NEAR/NearOn/WiggleFilter ==
  TuneTOP : Subsystem  mask(Talaria Trivial Tune TOP){TriggerInit=[-85 142 85 198], TopName=NearWiggleCoeffs, TuneName=NearWiggleCoeffs, DataTypeOut=single, MaskValue=Config.DefaultNearWiggleCoeffs, TunabilityNumber=1, MinValue=[], MaxValue=[], BankNumber=0, PreOverlay=false, PostOverlay=false, UseSameName=on}
      mask prompts: TriggerInit "Hidden: MoveFcn redraw"; TopName "Name:"; TuneName "Name of TuneVar:"; DataTypeOut "Data type:"; MaskValue "Default Value:"; TunabilityNumber "Tunability:"; MinValue "Min Value:"; MaxValue "Max Value:"; BankNumber "Target memory bank number:"; PreOverlay "Requires pre-overlay action:"; PostOverlay "Requires post-overlay action:"; UseSameName "Use same name for tune variable and TOP"
      mask help: The TuneTOP block encapsultes a Target Overlay Parameter, a Tune Variable, and a Trivial Translation between them.
      mask init:
      | [ok,activeTopPath,activeTunePath] = TuneTOP_Mask.Init(gcbh);
      settings: MoveFcn=TuneTOP_Mask.CB_TriggerInit(gcbh);
      mask Callback TriggerInit: TuneTOP_Mask.CB_TriggerInit(gcbh);
      mask TypeOptions TopName: TOP/TopName
      mask TypeOptions TuneName: Tune Variable/TuneName
      mask TypeOptions DataTypeOut: TOP/DataTypeOut
      mask TypeOptions MaskValue: Tune Variable/MaskValue
      mask TypeOptions TunabilityNumber: Tune Variable/TunabilityNumber
      mask Callback TunabilityNumber: TuneVarMask.CB_TunabilityNumber(gcbh);
      mask TypeOptions MinValue: Tune Variable/MinValue
      mask TypeOptions MaxValue: Tune Variable/MaxValue
      mask TypeOptions BankNumber: TOP/BankNumber
      mask TypeOptions PreOverlay: TOP/PreOverlay
      mask TypeOptions PostOverlay: TOP/PostOverlay
      mask Callback UseSameName: TuneTOP_Mask.CB_UseSameName(gcbh);
      mask DialogControl toolPanel Prompt: Tuning Tool Hints
      mask DialogControl DescriptionGroup Prompt: Description
      mask DialogControl EditDescription Prompt: Edit Description
      mask DialogControl EditDescription Callback: TuneTOP_Mask.CB_EditDescription(gcbh);
      mask DialogControl TunabilityText Prompt: Easy: Changes nearly every tuning.
      mask DialogControl AdvancedPanel Prompt: Advanced
      mask DialogControl ConvertToFullTranslation Prompt: Irreversible conversion to full translation
      mask DialogControl ConvertToFullTranslation Callback: TuneTOP_Mask.CB_ConvertToFullTranslation(gcbh);
      mask DialogControl ErrorContainer Prompt: Error Messages
      mask DialogControl ErrorText Prompt: Default value cannot be empty. Tune variables must have non-zero dimensions.
      mask Display:
      | % retrieve icon definition
      | [path,w,h] = TuneTOP_Mask.Icon();
      | 
      | % retrieve the block's pixel size
      | pos = get(gcbh,'position');
      | bw = pos(3) - pos(1);
      | bh = pos(4) - pos(2);
      | 
      | % draw centered icon
      | xAdj = bw/2 - w/2 + 5;
      | yAdj = bh/2 - h/2 + 4;
      | for i=1:length(path)
      | 	patch(path(i).x+xAdj, path(i).y+yAdj, path(i).rgb);
      | end
      | 
      | % show the top name or an X
      | if (exist('ok','var') && ok)
      | 	text(bw*0.5, bh*0.2, activeTopPath, 'horizontalAlignment', 'center');
      | 	patch(0,0,[1 1 1]);
      | 	patch(bw,bh,[1 1 1]);
      | else
      | 	tx=bw*0.03;
      | 	ty=bh*0.03;
      | 	patch([0 tx bw bw-tx], [ty 0 bh-ty bh], [1 0 0]);
      | 	patch([0 bw-tx bw tx], [bh-ty 0 ty bh], [1 0 0]);
      | end
  TuneTOP1 : Subsystem  mask(Talaria Trivial Tune TOP){TriggerInit=[130 -28 300 28], TopName=NearDelay, TuneName=NearDelay, DataTypeOut=single, MaskValue=Config.DefaultNearDelay, TunabilityNumber=1, MinValue=[], MaxValue=[], BankNumber=0, PreOverlay=false, PostOverlay=false, UseSameName=on}
      mask prompts: TriggerInit "Hidden: MoveFcn redraw"; TopName "Name:"; TuneName "Name of TuneVar:"; DataTypeOut "Data type:"; MaskValue "Default Value:"; TunabilityNumber "Tunability:"; MinValue "Min Value:"; MaxValue "Max Value:"; BankNumber "Target memory bank number:"; PreOverlay "Requires pre-overlay action:"; PostOverlay "Requires post-overlay action:"; UseSameName "Use same name for tune variable and TOP"
      mask help: The TuneTOP block encapsultes a Target Overlay Parameter, a Tune Variable, and a Trivial Translation between them.
      mask init:
      | [ok,activeTopPath,activeTunePath] = TuneTOP_Mask.Init(gcbh);
      settings: MoveFcn=TuneTOP_Mask.CB_TriggerInit(gcbh);
      mask Callback TriggerInit: TuneTOP_Mask.CB_TriggerInit(gcbh);
      mask TypeOptions TopName: TOP/TopName
      mask TypeOptions TuneName: Tune Variable/TuneName
      mask TypeOptions DataTypeOut: TOP/DataTypeOut
      mask TypeOptions MaskValue: Tune Variable/MaskValue
      mask TypeOptions TunabilityNumber: Tune Variable/TunabilityNumber
      mask Callback TunabilityNumber: TuneVarMask.CB_TunabilityNumber(gcbh);
      mask TypeOptions MinValue: Tune Variable/MinValue
      mask TypeOptions MaxValue: Tune Variable/MaxValue
      mask TypeOptions BankNumber: TOP/BankNumber
      mask TypeOptions PreOverlay: TOP/PreOverlay
      mask TypeOptions PostOverlay: TOP/PostOverlay
      mask Callback UseSameName: TuneTOP_Mask.CB_UseSameName(gcbh);
      mask DialogControl toolPanel Prompt: Tuning Tool Hints
      mask DialogControl DescriptionGroup Prompt: Description
      mask DialogControl EditDescription Prompt: Edit Description
      mask DialogControl EditDescription Callback: TuneTOP_Mask.CB_EditDescription(gcbh);
      mask DialogControl TunabilityText Prompt: Easy: Changes nearly every tuning.
      mask DialogControl AdvancedPanel Prompt: Advanced
      mask DialogControl ConvertToFullTranslation Prompt: Irreversible conversion to full translation
      mask DialogControl ConvertToFullTranslation Callback: TuneTOP_Mask.CB_ConvertToFullTranslation(gcbh);
      mask DialogControl ErrorContainer Prompt: Error Messages
      mask Display:
      | % retrieve icon definition
      | [path,w,h] = TuneTOP_Mask.Icon();
      | 
      | % retrieve the block's pixel size
      | pos = get(gcbh,'position');
      | bw = pos(3) - pos(1);
      | bh = pos(4) - pos(2);
      | 
      | % draw centered icon
      | xAdj = bw/2 - w/2 + 5;
      | yAdj = bh/2 - h/2 + 4;
      | for i=1:length(path)
      | 	patch(path(i).x+xAdj, path(i).y+yAdj, path(i).rgb);
      | end
      | 
      | % show the top name or an X
      | if (exist('ok','var') && ok)
      | 	text(bw*0.5, bh*0.2, activeTopPath, 'horizontalAlignment', 'center');
      | 	patch(0,0,[1 1 1]);
      | 	patch(bw,bh,[1 1 1]);
      | else
      | 	tx=bw*0.03;
      | 	ty=bh*0.03;
      | 	patch([0 tx bw bw-tx], [ty 0 bh-ty bh], [1 0 0]);
      | 	patch([0 bw-tx bw tx], [bh-ty 0 ty bh], [1 0 0]);
      | end

== system Model_TranslationEngine64/ModelPreAmp/DecRate/Medusa5H1/SleepingBeauty/SleepingBeauty/Enabled/FadeControl ==
  InnerLink : Subsystem  mask(Blocklib FadeControl){Config=InnerLinkConfig, FeatureName=FadeControl}
      mask prompts: Config "FadeControlConfig"; FeatureName "Feature path name:"
      mask help: This component is to be used in conjunction with 1 or more instances of the FadeRamper block. It provides the control layer for Fade processing via an RTC and tune variables.
      mask init:
      | blkh=gcbh;
      | Config=BTConfig.Assert(blkh,Config);
      | Config.Validate();
      | BTConfig.InitSetFeatureIfPresent(blkh,'FeatureName');
      | 
      | % Set boundary conditions
      | rampRateBounds = [5,50000];
      | rampTimeBounds = [1,3000];
      mask Help: If this control block is being used in a "multi-instance" manner, i.e. it is contorlling two or more FadeRamper blocks, there is an additional step that must be done. The developer must add a function-triggered subsytem containing an AND logic gate, which will combine the notification completion signals of the multiple ramper instances. The output of this subsytem must then feed the NTF_done input of the FadeControl block.
      mask Callback Config: BTConfig.CallbackHideIfPresent(gcbh,{'FeatureName'});
      mask TypeOptions FeatureName: FeaturePath/FeatureName

== system Model_TranslationEngine64/ModelPreAmp/DecRate/Medusa5H1/SleepingBeauty/SleepingBeauty/Enabled/FadeRamperDR ==
  InnerLink : Subsystem  mask(Blocklib FadeRamper){Config=InnerLinkConfig, FeatureName=FadeRamperDR, EnableGainOut=on}
      mask prompts: Config "FadeRamperConfig"; FeatureName "Feature path name:"; EnableGainOut "Enable gain output"
      mask help:
      | This component is to be used in conjunction with the FadeControl block, which provides runtime control and tuning capabilities. Multiple instances of this block may be placed within an audio application, and a single FadeControl block has the ability to control all of these rampers simultaneously.
      |
      | For "Instance Name", please enter a name for the block. For example, if this is one of multiple instances of FadeRamper, then name each block accordingly so that the subsequent tune variables will route correctly.
      |
      | i.e. FadeRamper1, FadeRamper2, FadeRamperFullRate, etc.
      mask init:
      | blkh=gcbh;
      | Config=BTConfig.Assert(blkh,Config);
      | Config.Validate();
      | BTConfig.InitSetFeatureIfPresent(blkh,'FeatureName');
      | 
      | % Mask initialization code (static-init DSMs, output ports)
      | FadeRamperMask.Init(blkh,EnableGainOut);
      mask Callback Config: BTConfig.CallbackHideIfPresent(gcbh,{'FeatureName'});
      mask TypeOptions FeatureName: FeaturePath/FeatureName

== system Model_TranslationEngine64/ModelPreAmp/DecRate/Medusa5H1/SleepingBeauty/SleepingBeauty/Enabled/FadeRamperFR ==
  InnerLink : Subsystem  mask(Blocklib FadeRamper){Config=InnerLinkConfig, FeatureName=FadeRamperFR, EnableGainOut=on}
      mask prompts: Config "FadeRamperConfig"; FeatureName "Feature path name:"; EnableGainOut "Enable gain output"
      mask help:
      | This component is to be used in conjunction with the FadeControl block, which provides runtime control and tuning capabilities. Multiple instances of this block may be placed within an audio application, and a single FadeControl block has the ability to control all of these rampers simultaneously.
      |
      | For "Instance Name", please enter a name for the block. For example, if this is one of multiple instances of FadeRamper, then name each block accordingly so that the subsequent tune variables will route correctly.
      |
      | i.e. FadeRamper1, FadeRamper2, FadeRamperFullRate, etc.
      mask init: same as Model_TranslationEngine64/ModelPreAmp/DecRate/Medusa5H1/SleepingBeauty/SleepingBeauty/Enabled/FadeRamperDR/InnerLink
      mask Callback Config: BTConfig.CallbackHideIfPresent(gcbh,{'FeatureName'});
      mask TypeOptions FeatureName: FeaturePath/FeatureName
